simulink model "Gripper_2Belts_solution"  (R2025b)
settings: Solver=ode23t  StartTime=0.0  StopTime=30  MaxStep=0.01  RelTol=1e-3  AbsTol=1e-4
StartFcn:
  | tic;
StopFcn:
  | Elapsed_Sim_Time = toc;
  | disp(['Elapsed Sim Time = ' num2str(Elapsed_Sim_Time)]);
model workspace (MATLAB code in the model file):
  | floor_l = 1.0900;
  | floor_d = 0.0100;
  | 
  | belt_w = 0.1000;
  | belt_l = 0.4000;
  | belt_h = 0.0200;
  | belt_in_offset = [0    0.5050 0.0500];
  | belt_out_offset = [-0.5050 0 0.0500];
  | belt_spd = 0.1;
  | 
  | cube_d = 0.0600;
  | cube_con_rsph = 0.003;
  | 
  | cube_con_k = 1000000;
  | cube_con_b = 10000;
  | 
  | finger_con_x = 0.01;
  | finger_con_y = 0.01;
  | finger_con_z = 5e-4;
  | finger_con_rsph = 5.0000e-04;
  | finger_con_muk = 0.05;
  | finger_con_mus = 0.07;
  | finger_con_vth = 1e-3;
  | 
  | finger_l = 0.4;
  | finger_w = 0.03;
  | finger_t = 0.01;
undefined symbols (not defined in the file): Extr_Data_LinkHoles, sigbuilder_block, X, Y, Z
libraries: sm_lib x47, fl_lib x16, nesl_utility x12, Parts_Lib x10, Contact_Forces_Lib x4, simulink x3, fl_ps_legacy_lib x1
(part 2 of 2)

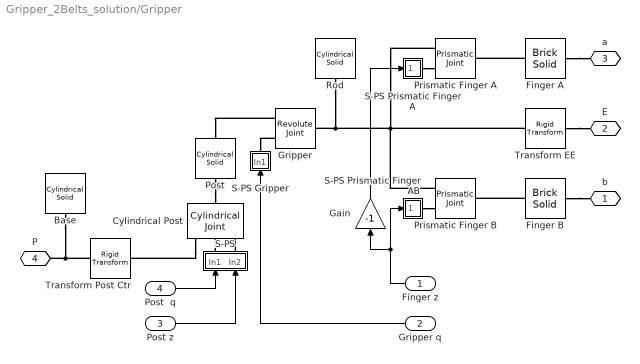
== system Gripper_2Belts_solution/Gripper ==
  Finger z : Inport
  Gripper q : Inport  Port=2
  Post z : Inport  Port=3
  Post  q : Inport  Port=4
  Base : sm_lib/Body Elements/Cylindrical Solid  CylinderRadius=0.03  CylinderRadiusUnits=m  CylinderLength=0.05  CylinderLengthUnits=m  ExportEntireGeometry=off  InertiaType=CalculateFromGeometry  BasedOnType=Density  Density=1000  DensityUnits=kg/m^3  Mass=1  MassUnits=kg  CenterOfMass=[0 0 0]  CenterOfMassUnits=m  MomentsOfInertia=[1 1 1]  MomentsOfInertiaUnits=kg*m^2  ProductsOfInertia=[1 1 1]  ProductsOfInertiaUnits=kg*m^2  GraphicType=FromGeometry  MarkerShape=Sphere  MarkerSize=10  GraphicVisPropType=SimpleVisualProperties  GraphicDiffuseColor=[0.5 0.5 0.5]  GraphicOpacity=1.0  GraphicSpecularColor=[0.5 0.5 0.5 1.0]  GraphicAmbientColor=[0.15 0.15 0.15 1.0]  GraphicEmissiveColor=[0.0 0.0 0.0 1.0]  GraphicShininess=75  DoExposeReferenceFrame=off  SerializedFrames=<Frames><Frame><Id>Frame1</Id><Value><Name>B</Name><Origin><Source>GeometricFeature</Source><FeatureName>bottom surface</FeatureName></Origin><PrimaryAxis><DefinedDirection>+Z</DefinedDirection><Source>ReferenceFrame</Source><SourceDirection>+Z</SourceDirection><FeatureName></FeatureName></PrimaryAxis><SecondaryAxis><DefinedDirection>+X</DefinedDirection><Source>ReferenceFrame</Source><SourceDirection>+X</SourceDirection><FeatureName></FeatureName></SecondaryAxis></Value></Frame></Frames>
  Cylindrical Post : sm_lib/Joints/Cylindrical Joint  JointMode=Normal  CompositeWrenchDir=FollowerOnBase  CompositeWrenchFrame=BaseFrame  SenseConstraintForce=off  SenseConstraintTorque=off  SenseTotalForce=off  SenseTotalTorque=off  RzPositionTargetSpecify=off  RzPositionTargetPriority=High  RzPositionTargetValue=0  RzPositionTargetValueUnits=deg  RzVelocityTargetSpecify=off  RzVelocityTargetPriority=High  RzVelocityTargetValue=0  RzVelocityTargetValueUnits=deg/s  RzEquilibriumPosition=0  RzEquilibriumPositionUnits=deg  RzSpringStiffness=0  RzSpringStiffnessUnits=N*m/deg  RzDampingCoefficient=0  RzDampingCoefficientUnits=N*m/(deg/s)  RzLowerLimitSpecify=off  RzLowerLimitBound=-90  RzLowerLimitBoundUnits=deg  RzLowerLimitStiffness=1e4  RzLowerLimitStiffnessUnits=N*m/deg  RzLowerLimitDamping=10  RzLowerLimitDampingUnits=N*m/(deg/s)  RzLowerLimitTransitionRegionWidth=0.1  RzLowerLimitTransitionRegionWidthUnits=deg  RzUpperLimitSpecify=off  RzUpperLimitBound=90  RzUpperLimitBoundUnits=deg  RzUpperLimitStiffness=1e4  RzUpperLimitStiffnessUnits=N*m/deg  RzUpperLimitDamping=10  RzUpperLimitDampingUnits=N*m/(deg/s)  RzUpperLimitTransitionRegionWidth=0.1  RzUpperLimitTransitionRegionWidthUnits=deg  RzTorqueActuationMode=ComputedTorque  RzMotionActuationMode=InputMotion  RzSensePosition=off  RzSenseVelocity=off  RzSenseAcceleration=off  RzSenseTorqueForce=off  RzSenseLowerLimitTorqueForce=off  RzSenseUpperLimitTorqueForce=off  PzPositionTargetSpecify=off  PzPositionTargetPriority=High  PzPositionTargetValue=0  PzPositionTargetValueUnits=m  PzVelocityTargetSpecify=off  PzVelocityTargetPriority=High  PzVelocityTargetValue=0  PzVelocityTargetValueUnits=m/s  PzEquilibriumPosition=0  PzEquilibriumPositionUnits=m  PzSpringStiffness=0  PzSpringStiffnessUnits=N/m  PzDampingCoefficient=0  PzDampingCoefficientUnits=N/(m/s)  PzLowerLimitSpecify=off  PzLowerLimitBound=-1  PzLowerLimitBoundUnits=m  PzLowerLimitStiffness=1e6  PzLowerLimitStiffnessUnits=N/m  PzLowerLimitDamping=1e3  PzLowerLimitDampingUnits=N/(m/s)  PzLowerLimitTransitionRegionWidth=1e-4  PzLowerLimitTransitionRegionWidthUnits=m  PzUpperLimitSpecify=off  PzUpperLimitBound=1  PzUpperLimitBoundUnits=m  PzUpperLimitStiffness=1e6  PzUpperLimitStiffnessUnits=N/m  PzUpperLimitDamping=1e3  PzUpperLimitDampingUnits=N/(m/s)  PzUpperLimitTransitionRegionWidth=1e-4  PzUpperLimitTransitionRegionWidthUnits=m  PzTorqueActuationMode=ComputedTorque  PzMotionActuationMode=InputMotion  PzSensePosition=off  PzSenseVelocity=off  PzSenseAcceleration=off  PzSenseTorqueForce=off  PzSenseLowerLimitTorqueForce=off  PzSenseUpperLimitTorqueForce=off
  Finger A : sm_lib/Body Elements/Brick Solid  BrickDimensions=[finger_t finger_l finger_w]  BrickDimensionsUnits=m  ExportEntireGeometry=off  InertiaType=CalculateFromGeometry  BasedOnType=Density  Density=1000  DensityUnits=kg/m^3  Mass=1  MassUnits=kg  CenterOfMass=[0 0 0]  CenterOfMassUnits=m  MomentsOfInertia=[1 1 1]  MomentsOfInertiaUnits=kg*m^2  ProductsOfInertia=[1 1 1]  ProductsOfInertiaUnits=kg*m^2  GraphicType=FromGeometry  MarkerShape=Sphere  MarkerSize=10  GraphicVisPropType=SimpleVisualProperties  GraphicDiffuseColor=[0.8 0.0 0.0]  GraphicOpacity=1.0  GraphicSpecularColor=[0.5 0.5 0.5 1.0]  GraphicAmbientColor=[0.15 0.15 0.15 1.0]  GraphicEmissiveColor=[0.0 0.0 0.0 1.0]  GraphicShininess=75  DoExposeReferenceFrame=off  SerializedFrames=<Frames><Frame><Id>Frame1</Id><Value><Name>Pr</Name><Origin><Source>GeometricFeature</Source><FeatureName>-y surface</FeatureName></Origin><PrimaryAxis><DefinedDirection>+Z</DefinedDirection><Source>ReferenceFrame</Source><SourceDirection>+X</SourceDirection><FeatureName></FeatureName></PrimaryAxis><SecondaryAxis><DefinedDirection>+X</DefinedDirection><Source>ReferenceFrame</Source><SourceDirection>+Y</SourceDirection><FeatureName></FeatureName></SecondaryAxis></Value></Frame><Frame><Id>Frame2</Id><Value><Name>G</Name><Origin><Source>GeometricFeature</Source><FeatureName>+x +y curve</FeatureName></Origin><PrimaryAxis><DefinedDirection>+Z</DefinedDirection><Source>ReferenceFrame</Source><SourceDirection>-X</SourceDirection><FeatureName></FeatureName></PrimaryAxis><SecondaryAxis><DefinedDirection>+X</DefinedDirection><Source>ReferenceFrame</Source><SourceDirection>-Z</SourceDirection><FeatureName></FeatureName></SecondaryAxis></Value></Frame></Frames>
  Finger B : sm_lib/Body Elements/Brick Solid  BrickDimensions=[finger_t finger_l finger_w]  BrickDimensionsUnits=m  ExportEntireGeometry=off  InertiaType=CalculateFromGeometry  BasedOnType=Density  Density=1000  DensityUnits=kg/m^3  Mass=1  MassUnits=kg  CenterOfMass=[0 0 0]  CenterOfMassUnits=m  MomentsOfInertia=[1 1 1]  MomentsOfInertiaUnits=kg*m^2  ProductsOfInertia=[1 1 1]  ProductsOfInertiaUnits=kg*m^2  GraphicType=FromGeometry  MarkerShape=Sphere  MarkerSize=10  GraphicVisPropType=SimpleVisualProperties  GraphicDiffuseColor=[0.8 0.0 0.0]  GraphicOpacity=1.0  GraphicSpecularColor=[0.5 0.5 0.5 1.0]  GraphicAmbientColor=[0.15 0.15 0.15 1.0]  GraphicEmissiveColor=[0.0 0.0 0.0 1.0]  GraphicShininess=75  DoExposeReferenceFrame=off  SerializedFrames=<Frames><Frame><Id>Frame1</Id><Value><Name>Pr</Name><Origin><Source>GeometricFeature</Source><FeatureName>-y surface</FeatureName></Origin><PrimaryAxis><DefinedDirection>+Z</DefinedDirection><Source>ReferenceFrame</Source><SourceDirection>+X</SourceDirection><FeatureName></FeatureName></PrimaryAxis><SecondaryAxis><DefinedDirection>+X</DefinedDirection><Source>ReferenceFrame</Source><SourceDirection>+Y</SourceDirection><FeatureName></FeatureName></SecondaryAxis></Value></Frame><Frame><Id>Frame2</Id><Value><Name>G</Name><Origin><Source>GeometricFeature</Source><FeatureName>-x +y curve</FeatureName></Origin><PrimaryAxis><DefinedDirection>+Z</DefinedDirection><Source>ReferenceFrame</Source><SourceDirection>+X</SourceDirection><FeatureName></FeatureName></PrimaryAxis><SecondaryAxis><DefinedDirection>+X</DefinedDirection><Source>ReferenceFrame</Source><SourceDirection>-Z</SourceDirection><FeatureName></FeatureName></SecondaryAxis></Value></Frame></Frames>
  Gain : Gain  Gain=-1
  Gripper : sm_lib/Joints/Revolute Joint  JointMode=Normal  CompositeWrenchDir=FollowerOnBase  CompositeWrenchFrame=BaseFrame  SenseConstraintForce=off  SenseConstraintTorque=off  SenseTotalForce=off  SenseTotalTorque=off  PositionTargetSpecify=off  PositionTargetPriority=High  PositionTargetValue=0  PositionTargetValueUnits=deg  VelocityTargetSpecify=off  VelocityTargetPriority=High  VelocityTargetValue=0  VelocityTargetValueUnits=deg/s  EquilibriumPosition=0  EquilibriumPositionUnits=deg  SpringStiffness=0  SpringStiffnessUnits=N*m/deg  DampingCoefficient=0  DampingCoefficientUnits=N*m/(deg/s)  LowerLimitSpecify=off  LowerLimitBound=-90  LowerLimitBoundUnits=deg  LowerLimitStiffness=1e4  LowerLimitStiffnessUnits=N*m/deg  LowerLimitDamping=10  LowerLimitDampingUnits=N*m/(deg/s)  LowerLimitTransitionRegionWidth=0.1  LowerLimitTransitionRegionWidthUnits=deg  UpperLimitSpecify=off  UpperLimitBound=90  UpperLimitBoundUnits=deg  UpperLimitStiffness=1e4  UpperLimitStiffnessUnits=N*m/deg  UpperLimitDamping=10  UpperLimitDampingUnits=N*m/(deg/s)  UpperLimitTransitionRegionWidth=0.1  UpperLimitTransitionRegionWidthUnits=deg  TorqueActuationMode=ComputedTorque  MotionActuationMode=InputMotion  SensePosition=off  SenseVelocity=off  SenseAcceleration=off  SenseTorqueForce=off  SenseLowerLimitTorqueForce=off  SenseUpperLimitTorqueForce=off
  Post : sm_lib/Body Elements/Cylindrical Solid  CylinderRadius=0.025  CylinderRadiusUnits=m  CylinderLength=0.1  CylinderLengthUnits=m  ExportEntireGeometry=off  InertiaType=CalculateFromGeometry  BasedOnType=Density  Density=1000  DensityUnits=kg/m^3  Mass=1  MassUnits=kg  CenterOfMass=[0 0 0]  CenterOfMassUnits=m  MomentsOfInertia=[1 1 1]  MomentsOfInertiaUnits=kg*m^2  ProductsOfInertia=[1 1 1]  ProductsOfInertiaUnits=kg*m^2  GraphicType=FromGeometry  MarkerShape=Sphere  MarkerSize=10  GraphicVisPropType=SimpleVisualProperties  GraphicDiffuseColor=[0.8 0.8 0.8]  GraphicOpacity=1.0  GraphicSpecularColor=[0.5 0.5 0.5 1.0]  GraphicAmbientColor=[0.15 0.15 0.15 1.0]  GraphicEmissiveColor=[0.0 0.0 0.0 1.0]  GraphicShininess=75  DoExposeReferenceFrame=on  SerializedFrames=<Frames><Frame><Id>Frame1</Id><Value><Name>Pr</Name><Origin><Source>GeometricFeature</Source><FeatureName>top surface</FeatureName></Origin><PrimaryAxis><DefinedDirection>+Z</DefinedDirection><Source>ReferenceFrame</Source><SourceDirection>+X</SourceDirection><FeatureName></FeatureName></PrimaryAxis><SecondaryAxis><DefinedDirection>+X</DefinedDirection><Source>ReferenceFrame</Source><SourceDirection>+Y</SourceDirection><FeatureName></FeatureName></SecondaryAxis></Value></Frame></Frames>
  Prismatic Finger A : sm_lib/Joints/Prismatic Joint  JointMode=Normal  CompositeWrenchDir=FollowerOnBase  CompositeWrenchFrame=BaseFrame  SenseConstraintForce=off  SenseConstraintTorque=off  SenseTotalForce=off  SenseTotalTorque=off  PositionTargetSpecify=off  PositionTargetPriority=High  PositionTargetValue=0  PositionTargetValueUnits=m  VelocityTargetSpecify=off  VelocityTargetPriority=High  VelocityTargetValue=0  VelocityTargetValueUnits=m/s  EquilibriumPosition=0  EquilibriumPositionUnits=m  SpringStiffness=0  SpringStiffnessUnits=N/m  DampingCoefficient=0  DampingCoefficientUnits=N/(m/s)  LowerLimitSpecify=off  LowerLimitBound=-1  LowerLimitBoundUnits=m  LowerLimitStiffness=1e6  LowerLimitStiffnessUnits=N/m  LowerLimitDamping=1e3  LowerLimitDampingUnits=N/(m/s)  LowerLimitTransitionRegionWidth=1e-4  LowerLimitTransitionRegionWidthUnits=m  UpperLimitSpecify=off  UpperLimitBound=1  UpperLimitBoundUnits=m  UpperLimitStiffness=1e6  UpperLimitStiffnessUnits=N/m  UpperLimitDamping=1e3  UpperLimitDampingUnits=N/(m/s)  UpperLimitTransitionRegionWidth=1e-4  UpperLimitTransitionRegionWidthUnits=m  TorqueActuationMode=ComputedTorque  MotionActuationMode=InputMotion  SensePosition=off  SenseVelocity=off  SenseAcceleration=off  SenseTorqueForce=off  SenseLowerLimitTorqueForce=off  SenseUpperLimitTorqueForce=off
  Prismatic Finger B : sm_lib/Joints/Prismatic Joint  JointMode=Normal  CompositeWrenchDir=FollowerOnBase  CompositeWrenchFrame=BaseFrame  SenseConstraintForce=off  SenseConstraintTorque=off  SenseTotalForce=off  SenseTotalTorque=off  PositionTargetSpecify=off  PositionTargetPriority=High  PositionTargetValue=0  PositionTargetValueUnits=m  VelocityTargetSpecify=off  VelocityTargetPriority=High  VelocityTargetValue=0  VelocityTargetValueUnits=m/s  EquilibriumPosition=0  EquilibriumPositionUnits=m  SpringStiffness=0  SpringStiffnessUnits=N/m  DampingCoefficient=0  DampingCoefficientUnits=N/(m/s)  LowerLimitSpecify=off  LowerLimitBound=-1  LowerLimitBoundUnits=m  LowerLimitStiffness=1e6  LowerLimitStiffnessUnits=N/m  LowerLimitDamping=1e3  LowerLimitDampingUnits=N/(m/s)  LowerLimitTransitionRegionWidth=1e-4  LowerLimitTransitionRegionWidthUnits=m  UpperLimitSpecify=off  UpperLimitBound=1  UpperLimitBoundUnits=m  UpperLimitStiffness=1e6  UpperLimitStiffnessUnits=N/m  UpperLimitDamping=1e3  UpperLimitDampingUnits=N/(m/s)  UpperLimitTransitionRegionWidth=1e-4  UpperLimitTransitionRegionWidthUnits=m  TorqueActuationMode=ComputedTorque  MotionActuationMode=InputMotion  SensePosition=off  SenseVelocity=off  SenseAcceleration=off  SenseTorqueForce=off  SenseLowerLimitTorqueForce=off  SenseUpperLimitTorqueForce=off
  Rod : sm_lib/Body Elements/Cylindrical Solid  CylinderRadius=0.01  CylinderRadiusUnits=m  CylinderLength=0.1  CylinderLengthUnits=m  ExportEntireGeometry=off  InertiaType=CalculateFromGeometry  BasedOnType=Density  Density=1000  DensityUnits=kg/m^3  Mass=1  MassUnits=kg  CenterOfMass=[0 0 0]  CenterOfMassUnits=m  MomentsOfInertia=[1 1 1]  MomentsOfInertiaUnits=kg*m^2  ProductsOfInertia=[1 1 1]  ProductsOfInertiaUnits=kg*m^2  GraphicType=FromGeometry  MarkerShape=Sphere  MarkerSize=10  GraphicVisPropType=SimpleVisualProperties  GraphicDiffuseColor=[0.0 0.4 0.6]  GraphicOpacity=1.0  GraphicSpecularColor=[0.5 0.5 0.5 1.0]  GraphicAmbientColor=[0.15 0.15 0.15 1.0]  GraphicEmissiveColor=[0.0 0.0 0.0 1.0]  GraphicShininess=75  DoExposeReferenceFrame=on  SerializedFrames=<Frames/>
  S-PS : Subsystem
      mask Display: disp('p, q')
  S-PS Gripper : Subsystem
      mask Display: disp('q')
  S-PS Prismatic Finger A : Subsystem
      mask Display: disp('p')
  S-PS Prismatic Finger AB : Subsystem
      mask Display: disp('p')
  Transform Post Ctr : sm_lib/Frames and Transforms/Rigid Transform  RotationMethod=None  FollAlignAxisA=+X  BaseAlignAxisA=+Y  FollAlignAxisB=+Y  BaseAlignAxisB=+Z  RotationStandardAxis=+Z  RotationAngle=0.0  RotationAngleUnits=deg  RotationArbitraryAxis=[0 0 1]  RotationSequenceAxes=FollowerAxes  RotationSequence=XYX  RotationSequenceAngles=[0 0 0]  RotationSequenceAnglesUnits=deg  RotationMatrix=[1 0 0; 0 1 0; 0 0 1]  Quaternion=[1 0 0 0]  TranslationMethod=StandardAxis  TranslationCartesianOffset=[0 0 0]  TranslationCartesianOffsetUnits=m  TranslationStandardAxis=+Z  TranslationStandardOffset=0.05  TranslationStandardOffsetUnits=m  TranslationROffset=0  TranslationROffsetUnits=m  TranslationThetaOffset=0  TranslationThetaOffsetUnits=deg  TranslationZOffset=0  TranslationZOffsetUnits=m
  Transform EE : sm_lib/Frames and Transforms/Rigid Transform  RotationMethod=None  FollAlignAxisA=+X  BaseAlignAxisA=+Y  FollAlignAxisB=+Y  BaseAlignAxisB=+Z  RotationStandardAxis=+Z  RotationAngle=0.0  RotationAngleUnits=deg  RotationArbitraryAxis=[0 0 1]  RotationSequenceAxes=FollowerAxes  RotationSequence=XYX  RotationSequenceAngles=[0 0 0]  RotationSequenceAnglesUnits=deg  RotationMatrix=[1 0 0; 0 1 0; 0 0 1]  Quaternion=[1 0 0 0]  TranslationMethod=StandardAxis  TranslationCartesianOffset=[0 0 0]  TranslationCartesianOffsetUnits=m  TranslationStandardAxis=+X  TranslationStandardOffset=finger_l-finger_w/2  TranslationStandardOffsetUnits=m  TranslationROffset=0  TranslationROffsetUnits=m  TranslationThetaOffset=0  TranslationThetaOffsetUnits=deg  TranslationZOffset=0  TranslationZOffsetUnits=m
  b : PMIOPort  Side=Right
  E : PMIOPort  Port=2  Side=Right
  a : PMIOPort  Port=3  Side=Right
  P : PMIOPort  Port=4  Side=Right
  wires:
  Finger z/1 -> Gain/1, S-PS Prismatic Finger AB/1(In1)
  Post  q/1 -> S-PS/1(In1)
  Post z/1 -> S-PS/2(In2)
  Gain/1 -> S-PS Prismatic Finger A/1(In1)
  Gripper q/1 -> S-PS Gripper/1(In1)
  connections:
  Finger B/RConn1 -- b/RConn1
  Finger A/RConn1 -- a/RConn1
  Gripper/LConn1 -- Post/LConn1
  Cylindrical Post/LConn1 -- Transform Post Ctr/RConn1
  Post/RConn1 -- Cylindrical Post/RConn1
  Prismatic Finger A/LConn1 -- Rod/RConn1 -- Gripper/RConn1 -- Transform EE/LConn1 -- Prismatic Finger B/LConn1
  S-PS Prismatic Finger AB/RConn1 -- Prismatic Finger B/LConn2
  S-PS/RConn1 -- Cylindrical Post/LConn2
  S-PS/RConn2 -- Cylindrical Post/LConn3
  S-PS Prismatic Finger A/RConn1 -- Prismatic Finger A/LConn2
  Gripper/LConn2 -- S-PS Gripper/RConn1
  Transform EE/RConn1 -- E/RConn1
  Transform Post Ctr/LConn1 -- Base/LConn1 -- P/RConn1
  Finger A/LConn1 -- Prismatic Finger A/RConn1
  Finger B/LConn1 -- Prismatic Finger B/RConn1

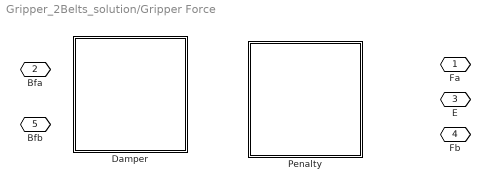
== system Gripper_2Belts_solution/Gripper Force ==
  Damper : Subsystem  VariantControl=Damper
  Penalty : Subsystem  VariantControl=Penalty
  Fa : PMIOPort  Side=Right
  Bfa : PMIOPort  Port=2  Side=Left
  E : PMIOPort  Port=3  Side=Right
  Fb : PMIOPort  Port=4  Side=Right
  Bfb : PMIOPort  Port=5  Side=Left

== system Gripper_2Belts_solution/Gripper/S-PS ==
  In1 : Inport
  In2 : Inport  Port=2
  Simulink-PS Converter2 : nesl_utility/Simulink-PS Converter  PhysicalDomain=network_engine_domain  SubClassName=ps_input  LeftPortType=input  RightPortType=output  PseudoPeriodic=off  Frequencies=[]  NoiseDistribution=none  NoiseParameters=[]  Unit=mm  AffineConversion=off  FilteringAndDerivatives=filter  SimscapeFilterOrder=2  InputFilterTimeConstant=0.005  UdotUserProvided=1
  Simulink-PS Converter3 : nesl_utility/Simulink-PS Converter  PhysicalDomain=network_engine_domain  SubClassName=ps_input  LeftPortType=input  RightPortType=output  PseudoPeriodic=off  Frequencies=[]  NoiseDistribution=none  NoiseParameters=[]  Unit=deg  AffineConversion=off  FilteringAndDerivatives=filter  SimscapeFilterOrder=2  InputFilterTimeConstant=0.005  UdotUserProvided=1
  Conn1 : PMIOPort  Side=Right
  Conn2 : PMIOPort  Port=2  Side=Right
  wires:
  In1/1 -> Simulink-PS Converter3/1
  In2/1 -> Simulink-PS Converter2/1
  connections:
  Simulink-PS Converter3/RConn1 -- Conn1/RConn1
  Simulink-PS Converter2/RConn1 -- Conn2/RConn1

== system Gripper_2Belts_solution/Gripper/S-PS Gripper ==
  In1 : Inport
  Simulink-PS Converter4 : nesl_utility/Simulink-PS Converter  PhysicalDomain=network_engine_domain  SubClassName=ps_input  LeftPortType=input  RightPortType=output  PseudoPeriodic=off  Frequencies=[]  NoiseDistribution=none  NoiseParameters=[]  Unit=deg  AffineConversion=off  FilteringAndDerivatives=filter  SimscapeFilterOrder=2  InputFilterTimeConstant=0.005  UdotUserProvided=1
  Conn1 : PMIOPort  Side=Right
  wires:
  In1/1 -> Simulink-PS Converter4/1
  connections:
  Conn1/RConn1 -- Simulink-PS Converter4/RConn1

== system Gripper_2Belts_solution/Gripper/S-PS Prismatic Finger A ==
  In1 : Inport
  Simulink-PS Converter1 : nesl_utility/Simulink-PS Converter  PhysicalDomain=network_engine_domain  SubClassName=ps_input  LeftPortType=input  RightPortType=output  PseudoPeriodic=off  Frequencies=[]  NoiseDistribution=none  NoiseParameters=[]  Unit=mm  AffineConversion=off  FilteringAndDerivatives=filter  SimscapeFilterOrder=2  InputFilterTimeConstant=0.005  UdotUserProvided=1
  Conn1 : PMIOPort  Side=Right
  wires:
  In1/1 -> Simulink-PS Converter1/1
  connections:
  Simulink-PS Converter1/RConn1 -- Conn1/RConn1

== system Gripper_2Belts_solution/Gripper/S-PS Prismatic Finger AB ==
  In1 : Inport
  Simulink-PS Converter1 : nesl_utility/Simulink-PS Converter  PhysicalDomain=network_engine_domain  SubClassName=ps_input  LeftPortType=input  RightPortType=output  PseudoPeriodic=off  Frequencies=[]  NoiseDistribution=none  NoiseParameters=[]  Unit=mm  AffineConversion=off  FilteringAndDerivatives=filter  SimscapeFilterOrder=2  InputFilterTimeConstant=0.005  UdotUserProvided=1
  Conn1 : PMIOPort  Side=Right
  wires:
  In1/1 -> Simulink-PS Converter1/1
  connections:
  Simulink-PS Converter1/RConn1 -- Conn1/RConn1

== system Gripper_2Belts_solution/Gripper Force/Damper ==
  Gripper Force : Subsystem  mask(Gripper Fingers to Load Force){cube_z=cube_d, contact_b=1e5, lpf_const_gripper_force=0.05, popup_relvel=Difference of relative velocities wrt. each finger}
      mask prompts: cube_z "Cube Length (m)"; contact_b "Damping Coefficient"; lpf_const_gripper_force "Low pass filter constant (s)"; popup_relvel "Load-gripper relative velocity along finger normal calculation:"
      mask help:
      | Models the force between the gripper fingers and the load as a controlled damper.  A very stiff 6-degree of freedom damping force becomes active when the load is between the fingers and the gripper fingers are closed enough to grasp the load.  This abstract method makes many assumptions about the interaction between the gripper and the load.
      |
      | Two options are provided to measure the velocity of the load normal to the gripper fingers.
      |
      | 1. Difference of relative velocity wrt. each finger
      | 2. Relative velocity wrt. gripper housing
      mask init:
      | temp_popup_relvel = get_param(gcb,'popup_relvel');
      | 
      | if (strncmpi(temp_popup_relvel,'Differ',6))
      |     set_param([gcb '/Relative vz'],'OverrideUsingVariant','Fingers');
      | else
      |     set_param([gcb '/Relative vz'],'OverrideUsingVariant','Housing');
      | end
      | 
      | clear temp_popup_relvel
      mask TypeOptions popup_relvel: Difference of relative velocities wrt. each finger | Relative velocity wrt. gripper housing
      mask DialogControl Container6 Prompt: Geometry
      mask DialogControl Container7 Prompt: Force
  Fa : PMIOPort  Side=Right
  Bfa : PMIOPort  Port=2  Side=Left
  E : PMIOPort  Port=3  Side=Right
  Fb : PMIOPort  Port=4  Side=Right
  Bfb : PMIOPort  Port=5  Side=Left
  connections:
  Gripper Force/RConn3 -- Fb/RConn1
  Gripper Force/RConn1 -- Fa/RConn1
  Gripper Force/LConn1 -- Bfb/RConn1
  E/RConn1 -- Gripper Force/RConn2

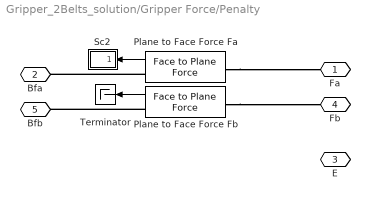
== system Gripper_2Belts_solution/Gripper Force/Penalty ==
  Plane to Face Force Fa : Contact_Forces_Lib/3D/Composite Forces/Face to Plane Force  PlaB_x=cube_d  PlaB_y=cube_d  PlaB_z=cube_d/2  FacF_x=finger_con_x  FacF_y=finger_con_y  FacF_z=finger_con_z  FacF_rSph=finger_con_rsph  force_law_pla2pla=Linear  k_contact_pla2pla=cube_con_k  b_contact_pla2pla=cube_con_b  pen_full_damp_F_pla2pla=1e-4  pen_exponent_pla2pla=1  friction_law_pla2pla=Stick-Slip Continuous  mu_kinetic_pla2pla=finger_con_muk  mu_static_pla2pla=finger_con_mus  v_thr_pla2pla=finger_con_vth  vis_on_pla2pla=off  vis_opc_en_box2box=0  vis_len_plaLz=0.0005  vis_clr=[0.9 0.2 0.2]  vis_opc=0.7
      settings: SourceProductName=Simscape Multibody Contact Forces Library
  Plane to Face Force Fb : Contact_Forces_Lib/3D/Composite Forces/Face to Plane Force  PlaB_x=cube_d  PlaB_y=cube_d  PlaB_z=cube_d/2  FacF_x=finger_con_x  FacF_y=finger_con_y  FacF_z=finger_con_z  FacF_rSph=finger_con_rsph  force_law_pla2pla=Linear  k_contact_pla2pla=cube_con_k  b_contact_pla2pla=cube_con_b  pen_full_damp_F_pla2pla=1e-4  pen_exponent_pla2pla=1  friction_law_pla2pla=Stick-Slip Continuous  mu_kinetic_pla2pla=finger_con_muk  mu_static_pla2pla=finger_con_mus  v_thr_pla2pla=finger_con_vth  vis_on_pla2pla=off  vis_opc_en_box2box=0  vis_len_plaLz=0.0005  vis_clr=[0.9 0.2 0.2]  vis_opc=0.7
      settings: SourceProductName=Simscape Multibody Contact Forces Library
  Sc2 : Subsystem
  Terminator : Terminator
  Fa : PMIOPort  Side=Right
  Bfa : PMIOPort  Port=2  Side=Left
  E : PMIOPort  Port=3  Side=Right
  Fb : PMIOPort  Port=4  Side=Right
  Bfb : PMIOPort  Port=5  Side=Left
  wires:
  Plane to Face Force Fa/1 -> Sc2/1(In1)
  Plane to Face Force Fb/1 -> Terminator/1
  connections:
  Plane to Face Force Fb/RConn1 -- Bfb/RConn1
  Plane to Face Force Fa/RConn1 -- Bfa/RConn1
  Plane to Face Force Fa/LConn1 -- Fa/RConn1
  Plane to Face Force Fb/LConn1 -- Fb/RConn1

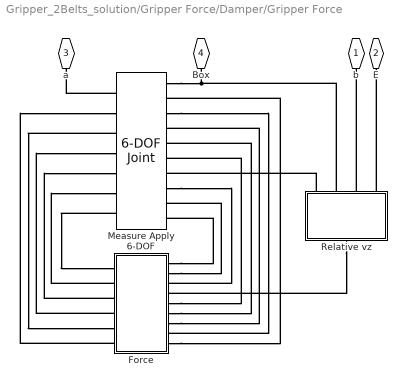
== system Gripper_2Belts_solution/Gripper Force/Damper/Gripper Force ==
  Force : Subsystem  mask(Controlled 6-DOF Damping Force){b=contact_b, lpfilt_const_force=lpf_const_gripper_force}
      mask prompts: b "Damping Coefficient"; lpfilt_const_force "Low Pass Filter Constant"
      mask help: Models a controlled 6-DOF damping force. If the distance between two frames is within a certain range (px, py, pz), the damping force is active.
  Measure Apply 6-DOF : sm_lib/Joints/6-DOF Joint  JointMode=Normal  CompositeWrenchDir=FollowerOnBase  CompositeWrenchFrame=BaseFrame  SenseConstraintForce=off  SenseConstraintTorque=off  SenseTotalForce=off  SenseTotalTorque=off  PxPositionTargetSpecify=off  PxPositionTargetPriority=High  PxPositionTargetValue=0  PxPositionTargetValueUnits=m  PxVelocityTargetSpecify=off  PxVelocityTargetPriority=High  PxVelocityTargetValue=0  PxVelocityTargetValueUnits=m/s  PxEquilibriumPosition=0  PxEquilibriumPositionUnits=m  PxSpringStiffness=0  PxSpringStiffnessUnits=N/m  PxDampingCoefficient=0  PxDampingCoefficientUnits=N/(m/s)  PxLowerLimitSpecify=off  PxLowerLimitBound=-1  PxLowerLimitBoundUnits=m  PxLowerLimitStiffness=1e6  PxLowerLimitStiffnessUnits=N/m  PxLowerLimitDamping=1e3  PxLowerLimitDampingUnits=N/(m/s)  PxLowerLimitTransitionRegionWidth=1e-4  PxLowerLimitTransitionRegionWidthUnits=m  PxUpperLimitSpecify=off  PxUpperLimitBound=1  PxUpperLimitBoundUnits=m  PxUpperLimitStiffness=1e6  PxUpperLimitStiffnessUnits=N/m  PxUpperLimitDamping=1e3  PxUpperLimitDampingUnits=N/(m/s)  PxUpperLimitTransitionRegionWidth=1e-4  PxUpperLimitTransitionRegionWidthUnits=m  PxTorqueActuationMode=InputTorque  PxMotionActuationMode=ComputedMotion  PxSensePosition=on  PxSenseVelocity=on  PxSenseAcceleration=off  PxSenseTorqueForce=off  PxSenseLowerLimitTorqueForce=off  PxSenseUpperLimitTorqueForce=off  PyPositionTargetSpecify=off  PyPositionTargetPriority=High  PyPositionTargetValue=40e-2  PyPositionTargetValueUnits=m  PyVelocityTargetSpecify=off  PyVelocityTargetPriority=High  PyVelocityTargetValue=0  PyVelocityTargetValueUnits=m/s  PyEquilibriumPosition=0  PyEquilibriumPositionUnits=m  PySpringStiffness=0  PySpringStiffnessUnits=N/m  PyDampingCoefficient=0  PyDampingCoefficientUnits=N/(m/s)  PyLowerLimitSpecify=off  PyLowerLimitBound=-1  PyLowerLimitBoundUnits=m  PyLowerLimitStiffness=1e6  PyLowerLimitStiffnessUnits=N/m  PyLowerLimitDamping=1e3  PyLowerLimitDampingUnits=N/(m/s)  PyLowerLimitTransitionRegionWidth=1e-4  PyLowerLimitTransitionRegionWidthUnits=m  PyUpperLimitSpecify=off  PyUpperLimitBound=1  PyUpperLimitBoundUnits=m  PyUpperLimitStiffness=1e6  PyUpperLimitStiffnessUnits=N/m  PyUpperLimitDamping=1e3  PyUpperLimitDampingUnits=N/(m/s)  PyUpperLimitTransitionRegionWidth=1e-4  PyUpperLimitTransitionRegionWidthUnits=m  PyTorqueActuationMode=InputTorque  PyMotionActuationMode=ComputedMotion  PySensePosition=on  PySenseVelocity=on  PySenseAcceleration=off  PySenseTorqueForce=off  PySenseLowerLimitTorqueForce=off  PySenseUpperLimitTorqueForce=off  PzPositionTargetSpecify=off  PzPositionTargetPriority=High  PzPositionTargetValue=0  PzPositionTargetValueUnits=m  PzVelocityTargetSpecify=off  PzVelocityTargetPriority=High  PzVelocityTargetValue=0  PzVelocityTargetValueUnits=m/s  PzEquilibriumPosition=0  PzEquilibriumPositionUnits=m  PzSpringStiffness=0  PzSpringStiffnessUnits=N/m  PzDampingCoefficient=0  PzDampingCoefficientUnits=N/(m/s)  PzLowerLimitSpecify=off  PzLowerLimitBound=-1  PzLowerLimitBoundUnits=m  PzLowerLimitStiffness=1e6  PzLowerLimitStiffnessUnits=N/m  PzLowerLimitDamping=1e3  PzLowerLimitDampingUnits=N/(m/s)  PzLowerLimitTransitionRegionWidth=1e-4  PzLowerLimitTransitionRegionWidthUnits=m  PzUpperLimitSpecify=off  PzUpperLimitBound=1  PzUpperLimitBoundUnits=m  PzUpperLimitStiffness=1e6  PzUpperLimitStiffnessUnits=N/m  PzUpperLimitDamping=1e3  PzUpperLimitDampingUnits=N/(m/s)  PzUpperLimitTransitionRegionWidth=1e-4  PzUpperLimitTransitionRegionWidthUnits=m  PzTorqueActuationMode=InputTorque  PzMotionActuationMode=ComputedMotion  PzSensePosition=on  PzSenseVelocity=on  PzSenseAcceleration=off  PzSenseTorqueForce=off  PzSenseLowerLimitTorqueForce=off  PzSenseUpperLimitTorqueForce=off  SphPositionTargetSpecify=off  SphPositionTargetPriority=High  SphPositionTargetRotationMethod=None  SphPositionTargetFollAlignAxisA=+X  SphPositionTargetBaseAlignAxisA=+Y  SphPositionTargetFollAlignAxisB=+Y  SphPositionTargetBaseAlignAxisB=+Z  SphPositionTargetRotationStandardAxis=+Z  SphPositionTargetRotationAngle=0.0  SphPositionTargetRotationAngleUnits=deg  SphPositionTargetRotationArbitraryAxis=[0 0 1]  SphPositionTargetRotationSequenceAxes=FollowerAxes  SphPositionTargetRotationSequence=XYX  SphPositionTargetRotationSequenceAngles=[0 0 0]  SphPositionTargetRotationSequenceAnglesUnits=deg  SphPositionTargetRotationMatrix=[1 0 0; 0 1 0; 0 0 1]  SphPositionTargetQuaternion=[1 0 0 0]  SphVelocityTargetSpecify=off  SphVelocityTargetPriority=High  SphVelocityTargetValue=[0 0 0]  SphVelocityTargetValueUnits=deg/s  SphVelocityTargetInFollowerFrame=on  SphEqPosRotationMethod=None  SphEqPosFollAlignAxisA=+X  SphEqPosBaseAlignAxisA=+Y  SphEqPosFollAlignAxisB=+Y  SphEqPosBaseAlignAxisB=+Z  SphEqPosRotationStandardAxis=+Z  SphEqPosRotationAngle=0.0  SphEqPosRotationAngleUnits=deg  SphEqPosRotationArbitraryAxis=[0 0 1]  SphEqPosRotationSequenceAxes=FollowerAxes  SphEqPosRotationSequence=XYX  SphEqPosRotationSequenceAngles=[0 0 0]  SphEqPosRotationSequenceAnglesUnits=deg  SphEqPosRotationMatrix=[1 0 0; 0 1 0; 0 0 1]  SphEqPosQuaternion=[1 0 0 0]  SphSpringStiffness=0  SphSpringStiffnessUnits=N*m/deg  SphDampingCoefficient=0  SphDampingCoefficientUnits=N*m/(deg/s)  SphLowerLimitSpecify=off  SphLowerLimitBound=15  SphLowerLimitBoundUnits=deg  SphLowerLimitStiffness=1e4  SphLowerLimitStiffnessUnits=N*m/deg  SphLowerLimitDamping=10  SphLowerLimitDampingUnits=N*m/(deg/s)  SphLowerLimitTransitionRegionWidth=0.1  SphLowerLimitTransitionRegionWidthUnits=deg  SphUpperLimitSpecify=off  SphUpperLimitBound=45  SphUpperLimitBoundUnits=deg  SphUpperLimitStiffness=1e4  SphUpperLimitStiffnessUnits=N*m/deg  SphUpperLimitDamping=10  SphUpperLimitDampingUnits=N*m/(deg/s)  SphUpperLimitTransitionRegionWidth=0.1  SphUpperLimitTransitionRegionWidthUnits=deg  SphTorqueActuationMode=InputTorque  SphActuateTorqueX=on  SphActuateTorqueY=on  SphActuateTorqueZ=on  SphActuateTorque=off  SphActuationFrame=BaseFrame  SphSensePosition=off  SphSenseVelocityX=on  SphSenseVelocityY=on  SphSenseVelocityZ=on  SphSenseVelocity=off  SphSenseAccelerationX=off  SphSenseAccelerationY=off  SphSenseAccelerationZ=off  SphSenseAcceleration=off  SphSenseLowerLimitTorqueMag=off  SphSenseUpperLimitTorqueMag=off  SphSensingFrame=BaseFrame
  Relative vz : Subsystem  Variant=on  VariantControlMode=label  LabelModeActiveChoice=Fingers
      settings: AttributesFormatString=%<ActiveVariant>
  b : PMIOPort  Side=Right
  E : PMIOPort  Port=2  Side=Right
  a : PMIOPort  Port=3  Side=Right
  Box : PMIOPort  Port=4  Side=Left
  connections:
  Force/LConn9 -- Measure Apply 6-DOF/RConn2
  Force/LConn7 -- Measure Apply 6-DOF/RConn4
  Force/LConn5 -- Measure Apply 6-DOF/RConn6
  Force/RConn4 -- Measure Apply 6-DOF/LConn4
  Force/LConn2 -- Measure Apply 6-DOF/RConn9
  Measure Apply 6-DOF/RConn8 -- Force/LConn3
  Force/RConn2 -- Measure Apply 6-DOF/LConn6
  Force/RConn3 -- Measure Apply 6-DOF/LConn5
  Force/RConn6 -- Measure Apply 6-DOF/LConn2
  Measure Apply 6-DOF/LConn3 -- Force/RConn5
  Measure Apply 6-DOF/RConn3 -- Force/LConn8
  Force/LConn6 -- Measure Apply 6-DOF/RConn5
  Force/LConn1 -- Measure Apply 6-DOF/RConn10
  Measure Apply 6-DOF/LConn1 -- a/RConn1
  Measure Apply 6-DOF/RConn1 -- Relative vz/LConn2 -- Box/RConn1
  Measure Apply 6-DOF/LConn7 -- Force/RConn1
  Relative vz/LConn3 -- b/RConn1
  Relative vz/LConn4 -- E/RConn1
  Relative vz/LConn1 -- Measure Apply 6-DOF/RConn7
  Relative vz/RConn1 -- Force/LConn4

== system Gripper_2Belts_solution/Gripper Force/Penalty/Sc2 ==
  In1 : Inport
  Bus Selector1 : BusSelector  OutputSignals=fz1.Normal Force,fz1.Friction Force,fz2.Normal Force,fz2.Friction Force,fz3.Normal Force,fz3.Friction Force,fz4.Normal Force,fz4.Friction Force
  Scope1 : Scope  NumInputPorts=8
      settings: ActiveDisplayYMinimum=-312.6734  ActiveDisplayYMaximum=2814.06064  DataLoggingVariableName=ScopeData2
  wires:
  Bus Selector1/8 -> Scope1/8  "<Friction Force>"
  Bus Selector1/7 -> Scope1/7  "<Normal Force>"
  Bus Selector1/5 -> Scope1/5  "<Normal Force>"
  In1/1 -> Bus Selector1/1
  Bus Selector1/6 -> Scope1/6  "<Friction Force>"
  Bus Selector1/2 -> Scope1/2  "<Friction Force>"
  Bus Selector1/4 -> Scope1/4  "<Friction Force>"
  Bus Selector1/3 -> Scope1/3  "<Normal Force>"
  Bus Selector1/1 -> Scope1/1  "<Normal Force>"

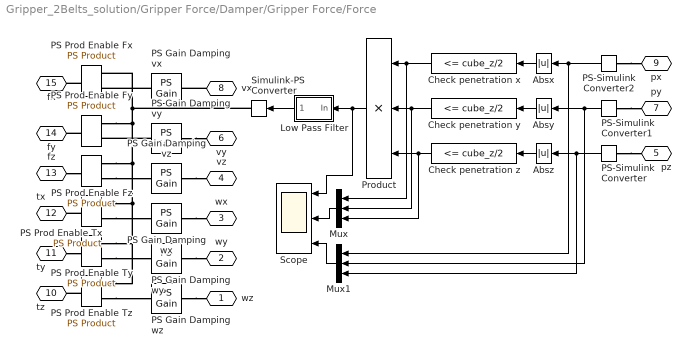
== system Gripper_2Belts_solution/Gripper Force/Damper/Gripper Force/Force ==
  Absx : Abs  ZeroCross=off  SaturateOnIntegerOverflow=off
  Absy : Abs  ZeroCross=off  SaturateOnIntegerOverflow=off
  Absz : Abs  ZeroCross=off  SaturateOnIntegerOverflow=off
  Check penetration x : simulink/Logic and Bit Operations/Compare To Constant  relop=<=  const=cube_z/2  OutDataTypeStr=boolean  ZeroCross=off
  Check penetration y : simulink/Logic and Bit Operations/Compare To Constant  relop=<=  const=cube_z/2  OutDataTypeStr=boolean  ZeroCross=off
  Check penetration z : simulink/Logic and Bit Operations/Compare To Constant  relop=<=  const=cube_z/2  OutDataTypeStr=boolean  ZeroCross=off
  Low Pass Filter : Subsystem  mask(First-order lag supporting vector signals){b=lpfilt_const_force, x_initial=0}
      mask prompts: b "Filter time constant"; x_initial "Initial output"
      mask help: Models a lag of the form 1/(b*s+1) where s is the Laplace operator.
  Mux : Mux  Inputs=3
  Mux1 : Mux  Inputs=3
  PS Gain Damping vx : fl_lib/Physical Signals/Functions/PS Gain  gain=-contact_b N/(m/s)
  PS Gain Damping vy : fl_lib/Physical Signals/Functions/PS Gain  gain=-contact_b N/(m/s)
  PS Gain Damping vz : fl_lib/Physical Signals/Functions/PS Gain  gain=-contact_b N/(m/s)
  PS Gain Damping wx : fl_lib/Physical Signals/Functions/PS Gain  gain=-contact_b N*m/(rad/s)
  PS Gain Damping wy : fl_lib/Physical Signals/Functions/PS Gain  gain=-contact_b N*m/(rad/s)
  PS Gain Damping wz : fl_lib/Physical Signals/Functions/PS Gain  gain=-contact_b N*m/(rad/s)
  PS Prod Enable Fx : fl_lib/Physical Signals/Functions/PS Product
  PS Prod Enable Fy : fl_lib/Physical Signals/Functions/PS Product
  PS Prod Enable Fz : fl_lib/Physical Signals/Functions/PS Product
  PS Prod Enable Tx : fl_lib/Physical Signals/Functions/PS Product
  PS Prod Enable Ty : fl_lib/Physical Signals/Functions/PS Product
  PS Prod Enable Tz : fl_lib/Physical Signals/Functions/PS Product
  PS-Simulink Converter : nesl_utility/PS-Simulink Converter  PhysicalDomain=network_engine_domain  SubClassName=ps_output  LeftPortType=input  RightPortType=output  PseudoPeriodic=off  Frequencies=[]  VectorFormat=1-D array  Unit=1  AffineConversion=off
  PS-Simulink Converter1 : nesl_utility/PS-Simulink Converter  PhysicalDomain=network_engine_domain  SubClassName=ps_output  LeftPortType=input  RightPortType=output  PseudoPeriodic=off  Frequencies=[]  VectorFormat=1-D array  Unit=1  AffineConversion=off
  PS-Simulink Converter2 : nesl_utility/PS-Simulink Converter  PhysicalDomain=network_engine_domain  SubClassName=ps_output  LeftPortType=input  RightPortType=output  PseudoPeriodic=off  Frequencies=[]  VectorFormat=1-D array  Unit=1  AffineConversion=off
  Product : Product  Inputs=3  OutDataTypeStr=double
  Scope : Scope  NumInputPorts=3
      settings: ActiveDisplayYMinimum=-0.125  ActiveDisplayYMaximum=1.125
  Simulink-PS Converter : nesl_utility/Simulink-PS Converter  PhysicalDomain=network_engine_domain  SubClassName=ps_input  LeftPortType=input  RightPortType=output  PseudoPeriodic=off  Frequencies=[]  NoiseDistribution=none  NoiseParameters=[]  Unit=1  AffineConversion=off  FilteringAndDerivatives=zero  SimscapeFilterOrder=1  InputFilterTimeConstant=0.005  UdotUserProvided=1
  wz : PMIOPort  Side=Left
  wy : PMIOPort  Port=2  Side=Left
  wx : PMIOPort  Port=3  Side=Left
  vz : PMIOPort  Port=4  Side=Left
  pz : PMIOPort  Port=5  Side=Left
  vy : PMIOPort  Port=6  Side=Left
  py : PMIOPort  Port=7  Side=Left
  vx : PMIOPort  Port=8  Side=Left
  px : PMIOPort  Port=9  Side=Left
  tz : PMIOPort  Port=10  Side=Right
  ty : PMIOPort  Port=11  Side=Right
  tx : PMIOPort  Port=12  Side=Right
  fz : PMIOPort  Port=13  Side=Right
  fy : PMIOPort  Port=14  Side=Right
  fx : PMIOPort  Port=15  Side=Right
  wires:
  PS-Simulink Converter1/1 -> Absy/1, Mux1/2
  PS-Simulink Converter2/1 -> Mux1/1, Absx/1
  Check penetration x/1 -> Mux/1, Product/1
  Check penetration y/1 -> Mux/2, Product/2
  Check penetration z/1 -> Mux/3, Product/3
  Mux/1 -> Scope/2
  Mux1/1 -> Scope/3
  PS-Simulink Converter/1 -> Mux1/3, Absz/1
  Absx/1 -> Check penetration x/1
  Absy/1 -> Check penetration y/1
  Absz/1 -> Check penetration z/1
  Product/1 -> Scope/1, Low Pass Filter/1(In)
  Low Pass Filter/1(Out) -> Simulink-PS Converter/1
  connections:
  vx/RConn1 -- PS Gain Damping vx/LConn1
  PS Gain Damping vx/RConn1 -- PS Prod Enable Fx/LConn2
  PS Gain Damping vy/RConn1 -- PS Prod Enable Fy/LConn2
  PS Gain Damping vy/LConn1 -- vy/RConn1
  PS Gain Damping vz/LConn1 -- vz/RConn1
  PS Prod Enable Fz/LConn2 -- PS Gain Damping vz/RConn1
  PS Prod Enable Tx/LConn2 -- PS Gain Damping wx/RConn1
  PS Gain Damping wx/LConn1 -- wx/RConn1
  PS Prod Enable Ty/LConn2 -- PS Gain Damping wy/RConn1
  PS Gain Damping wy/LConn1 -- wy/RConn1
  PS Prod Enable Tz/LConn2 -- PS Gain Damping wz/RConn1
  PS Gain Damping wz/LConn1 -- wz/RConn1
  PS-Simulink Converter/LConn1 -- pz/RConn1
  PS-Simulink Converter1/LConn1 -- py/RConn1
  PS-Simulink Converter2/LConn1 -- px/RConn1
  PS Prod Enable Tx/LConn1 -- PS Prod Enable Tz/LConn1 -- PS Prod Enable Ty/LConn1 -- PS Prod Enable Fz/LConn1 -- PS Prod Enable Fy/LConn1 -- PS Prod Enable Fx/LConn1 -- Simulink-PS Converter/RConn1
  PS Prod Enable Fx/RConn1 -- fx/RConn1
  PS Prod Enable Tz/RConn1 -- tz/RConn1
  ty/RConn1 -- PS Prod Enable Ty/RConn1
  PS Prod Enable Tx/RConn1 -- tx/RConn1
  fz/RConn1 -- PS Prod Enable Fz/RConn1
  PS Prod Enable Fy/RConn1 -- fy/RConn1

== system Gripper_2Belts_solution/Gripper Force/Damper/Gripper Force/Relative vz ==
  Fingers : Subsystem  VariantControl=Fingers
  Housing : Subsystem  VariantControl=Housing
  vz fa : PMIOPort  Side=Left
  Box : PMIOPort  Port=2  Side=Left
  b : PMIOPort  Port=3  Side=Left
  E : PMIOPort  Port=4  Side=Left
  vz : PMIOPort  Port=5  Side=Right

== system Gripper_2Belts_solution/Gripper Force/Damper/Gripper Force/Force/Low Pass Filter ==
  In : Inport
  Gain : Gain  Gain=1./b
  Integrator : Integrator  InitialCondition=x_initial.*b
  Sum : Sum  Inputs=|+-  InputSameDT=on  SaturateOnIntegerOverflow=on  OutDataTypeStr=Inherit: Same as first input
  Out : Outport  VectorParamsAs1DForOutWhenUnconnected=off
  wires:
  Sum/1 -> Integrator/1
  In/1 -> Sum/1
  Integrator/1 -> Gain/1
  Gain/1 -> Sum/2, Out/1

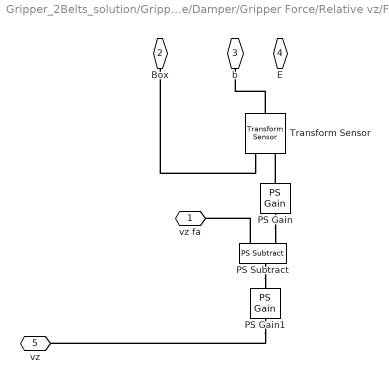
== system Gripper_2Belts_solution/Gripper Force/Damper/Gripper Force/Relative vz/Fingers ==
  PS Gain : fl_lib/Physical Signals/Functions/PS Gain  gain=1
  PS Gain1 : fl_lib/Physical Signals/Functions/PS Gain  gain=1
  PS Subtract : fl_lib/Physical Signals/Functions/PS Subtract
  Transform Sensor : sm_lib/Frames and Transforms/Transform Sensor  MeasurementFrame=Base  RotationSequence=XYX  SenseAngle=off  SenseAxis=off  SenseQ=off  SenseR=off  SenseRotationSequence=off  SenseOmegaX=off  SenseOmegaY=off  SenseOmegaZ=off  SenseOmega=off  SenseQDot=off  SenseRDot=off  SenseRotationSequenceDot=off  SenseAlphaX=off  SenseAlphaY=off  SenseAlphaZ=off  SenseAlpha=off  SenseQDDot=off  SenseRDDot=off  SenseX=off  SenseY=off  SenseZ=off  SenseXYZ=off  SenseRad=off  SenseAzim=off  SenseDist=off  SenseInc=off  SenseXDot=off  SenseYDot=off  SenseZDot=on  SenseXYZDot=off  SenseRadDot=off  SenseAzimDot=off  SenseDistDot=off  SenseIncDot=off  SenseXDDot=off  SenseYDDot=off  SenseZDDot=off  SenseXYZDDot=off  SenseRadDDot=off  SenseAzimDDot=off  SenseDistDDot=off  SenseIncDDot=off
  vz fa : PMIOPort  Side=Left
  Box : PMIOPort  Port=2  Side=Left
  b : PMIOPort  Port=3  Side=Left
  E : PMIOPort  Port=4  Side=Left
  vz : PMIOPort  Port=5  Side=Right
  connections:
  PS Subtract/LConn1 -- vz fa/RConn1
  PS Gain/LConn1 -- Transform Sensor/RConn2
  Transform Sensor/LConn1 -- b/RConn1
  PS Subtract/RConn1 -- PS Gain1/LConn1
  PS Gain/RConn1 -- PS Subtract/LConn2
  Transform Sensor/RConn1 -- Box/RConn1
  PS Gain1/RConn1 -- vz/RConn1

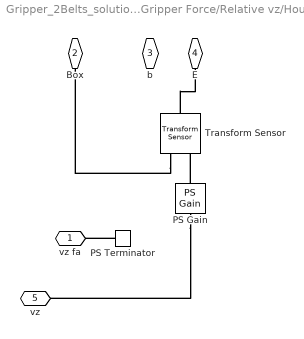
== system Gripper_2Belts_solution/Gripper Force/Damper/Gripper Force/Relative vz/Housing ==
  PS Gain : fl_ps_legacy_lib/Legacy Physical Signals/Functions/PS Gain  gain=-1
  PS Terminator : fl_lib/Physical Signals/Sinks/PS Terminator
  Transform Sensor : sm_lib/Frames and Transforms/Transform Sensor  MeasurementFrame=Base  RotationSequence=XYX  SenseAngle=off  SenseAxis=off  SenseQ=off  SenseR=off  SenseRotationSequence=off  SenseOmegaX=off  SenseOmegaY=off  SenseOmegaZ=off  SenseOmega=off  SenseQDot=off  SenseRDot=off  SenseRotationSequenceDot=off  SenseAlphaX=off  SenseAlphaY=off  SenseAlphaZ=off  SenseAlpha=off  SenseQDDot=off  SenseRDDot=off  SenseX=off  SenseY=off  SenseZ=off  SenseXYZ=off  SenseRad=off  SenseAzim=off  SenseDist=off  SenseInc=off  SenseXDot=off  SenseYDot=off  SenseZDot=on  SenseXYZDot=off  SenseRadDot=off  SenseAzimDot=off  SenseDistDot=off  SenseIncDot=off  SenseXDDot=off  SenseYDDot=off  SenseZDDot=off  SenseXYZDDot=off  SenseRadDDot=off  SenseAzimDDot=off  SenseDistDDot=off  SenseIncDDot=off
  vz fa : PMIOPort  Side=Left
  Box : PMIOPort  Port=2  Side=Left
  b : PMIOPort  Port=3  Side=Left
  E : PMIOPort  Port=4  Side=Left
  vz : PMIOPort  Port=5  Side=Right
  connections:
  Transform Sensor/RConn1 -- Box/RConn1
  PS Gain/RConn1 -- vz/RConn1
  Transform Sensor/LConn1 -- E/RConn1
  PS Gain/LConn1 -- Transform Sensor/RConn2
  PS Terminator/LConn1 -- vz fa/RConn1
